simulink model "longitudinal"  (R2019a)
settings: Solver=ode45  StartTime=0.0  StopTime=10  RelTol=1e-3
values from neighbouring files (symbols this model uses):
  I = 1.5    [LongAccParams.m]
  R_w = 0.32    [Fx_calculator.m]
undefined symbols (not defined in the file or in its folder): Ml
libraries: simulink x1
settings Model: Creator=afathaza  LastModifiedBy=a33shahi
settings SolverCC: ZeroCrossAlgorithm=Adaptive
settings DebuggingCC: IgnoredZcDiagnostic=none

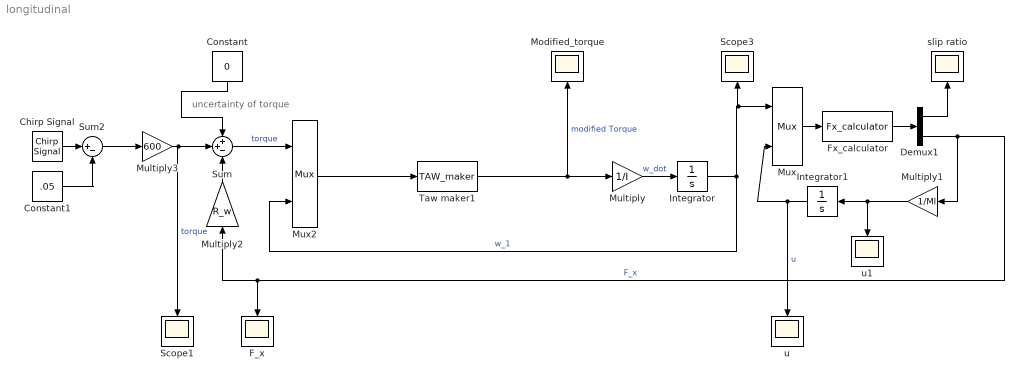
== system longitudinal ==
  note: uncertainty of torque
  Chirp Signal : simulink/Sources/Chirp Signal  f1=0.04  T=200  f2=.1
  Constant : Constant  Value=0
  Constant1 : Constant  Value=.05
  Demux1 : Demux  Outputs=2
  F_x : Scope
  Fx_calculator : MATLABFcn  MATLABFcn=Fx_calculator
  Integrator : Integrator  InitialCondition=0.12
  Integrator1 : Integrator  InitialCondition=0.1*R_w
  Modified_torque : Scope
  Multiply : Gain  Gain=1/I
  Multiply1 : Gain  Gain=1/Ml
  Multiply2 : Gain  Gain=R_w
  Multiply3 : Gain  Gain=600
  Mux : Mux  Inputs=2
      settings: DisplayOption=signals
  Mux2 : Mux  Inputs=2
      settings: DisplayOption=signals
  Scope1 : Scope
  Scope3 : Scope
  Sum : Sum  Inputs=++-
  Sum2 : Sum  Inputs=|+-
  Taw maker1 : MATLABFcn  MATLABFcn=TAW_maker
  slip ratio : Scope
  u : Scope
  u1 : Scope
  wires:
  Multiply2/1 -> Sum/3
  Constant1/1 -> Sum2/2
  Integrator1/1 -> Mux/2, u/1  "u"
  Sum2/1 -> Multiply3/1
  Chirp Signal/1 -> Sum2/1
  Multiply1/1 -> u1/1, Integrator1/1
  Mux/1 -> Fx_calculator/1
  Multiply/1 -> Integrator/1  "w_dot"
  Constant/1 -> Sum/1
  Multiply3/1 -> Scope1/1, Sum/2  "torque"
  Fx_calculator/1 -> Demux1/1
  Demux1/2 -> Multiply2/1, F_x/1, Multiply1/1  "F_x"
  Demux1/1 -> slip ratio/1
  Mux2/1 -> Taw maker1/1
  Sum/1 -> Mux2/1  "torque"
  Integrator/1 -> Scope3/1, Mux/1, Mux2/2  "w_1"
  Taw maker1/1 -> Multiply/1, Modified_torque/1  "modified Torque"
